simulink model "arna.slx"  (R2018b)
settings: Solver=VariableStepAuto  StartTime=0.0  StopTime=10.0  RelTol=1e-3
undefined symbols (not defined in the file or in its folder): B, F, K, M
settings Model: Creator=student  LastModifiedBy=student

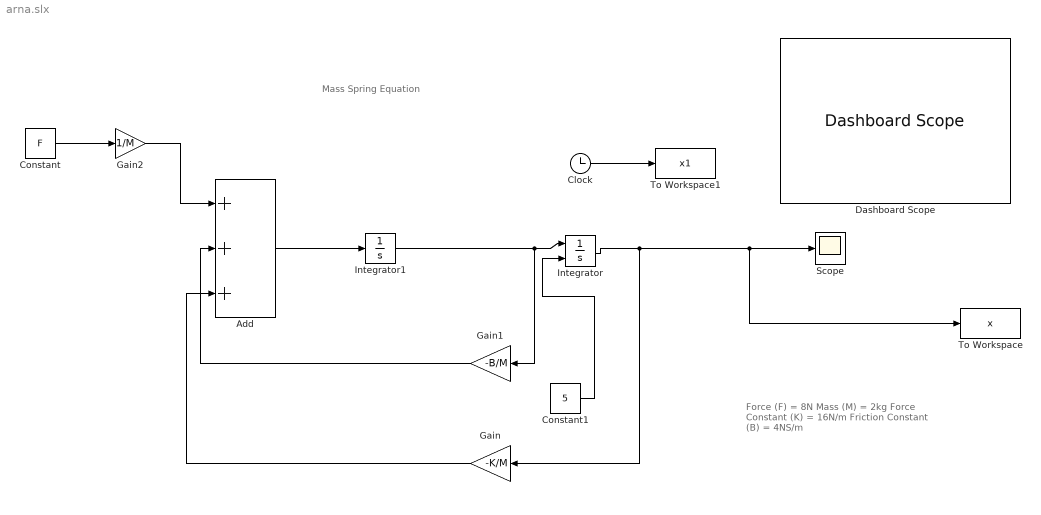
== system arna.slx ==
  note: Mass Spring Equation
  note: Force (F) = 8N
      | Mass (M) = 2kg
      | Force Constant (K) = 16N/m
      | Friction Constant (B) = 4NS/m
  Add : Sum  Inputs=+++
  Clock : Clock
  Constant : Constant  Value=F
  Constant1 : Constant  Value=5
  Dashboard Scope : DashboardScope  WebBlockId=15
  Gain : Gain  Gain=-K/M
  Gain1 : Gain  Gain=-B/M
  Gain2 : Gain  Gain=1/M
  Integrator : Integrator  InitialConditionSource=external
  Integrator1 : Integrator
  Scope : Scope
  To Workspace : ToWorkspace  VariableName=x  SampleTime=-1
  To Workspace1 : ToWorkspace  VariableName=x1  SampleTime=-1
  wires:
  Constant/1 -> Gain2/1
  Gain2/1 -> Add/1
  Add/1 -> Integrator1/1
  Integrator1/1 -> Gain1/1, Integrator/1
  Integrator/1 -> Gain/1, To Workspace/1, Scope/1
  Gain1/1 -> Add/2
  Gain/1 -> Add/3
  Constant1/1 -> Integrator/2
  Clock/1 -> To Workspace1/1
